simulink model "modeloProcessoAula4"  (R2022a)
settings: Solver=VariableStepAuto  StartTime=0.0  StopTime=400.0  RelTol=1e-3
values from neighbouring files (symbols this model uses):
  C = -14.405*(s + 0.0362)/s    [script.m]
  u0 = 52433    [script.m]
  y0 = 40982    [script.m]
libraries: cstblocks x5, slpidlib x1
settings Model: Creator=Victor  LastModifiedBy=Notebook_Artur
settings SolverCC: AlgebraicLoopSolver=TrustRegion
settings DebuggingCC: UnconnectedInputMsg=warning  UnconnectedOutputMsg=warning  UnconnectedLineMsg=warning  SFMachineParentedDataDiag=warning
settings RTWCC: DLArmComputeVersion=19.05

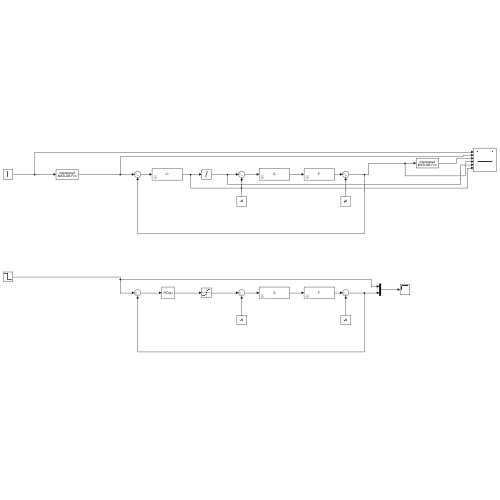
[thumbnail: Simulink's stored preview of the top-level diagram]
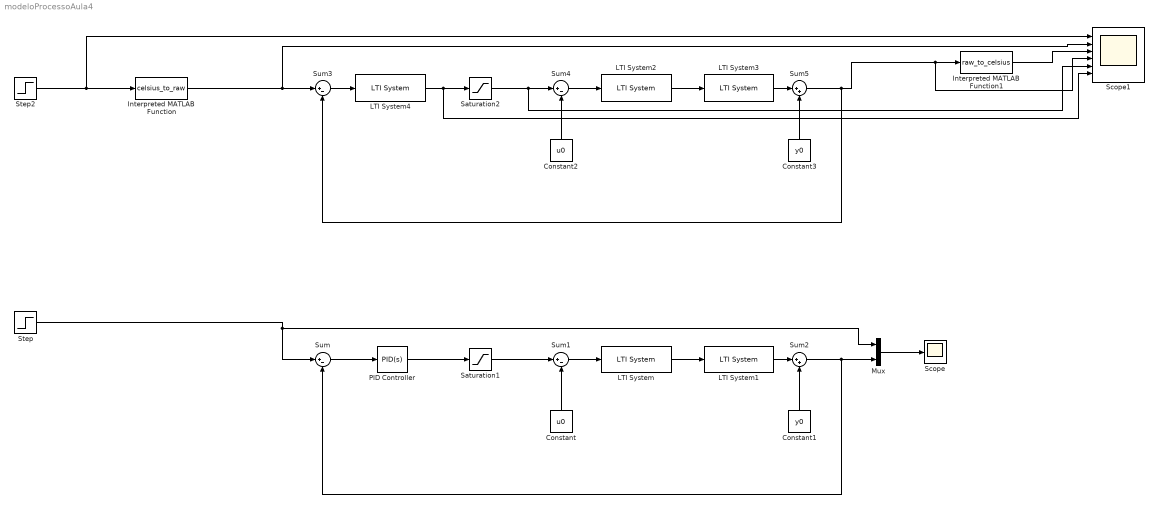
== system modeloProcessoAula4 ==
  Constant : Constant  Value=u0
  Constant1 : Constant  Value=y0
  Constant2 : Constant  Value=u0
  Constant3 : Constant  Value=y0
  Interpreted MATLAB Function : MATLABFcn  MATLABFcn=celsius_to_raw
  Interpreted MATLAB Function1 : MATLABFcn  MATLABFcn=raw_to_celsius
  LTI System : cstblocks/LTI System  sys=G  IC=[]
  LTI System1 : cstblocks/LTI System  sys=F  IC=[]
  LTI System2 : cstblocks/LTI System  sys=G  IC=[]
  LTI System3 : cstblocks/LTI System  sys=F  IC=[]
  LTI System4 : cstblocks/LTI System  sys=-C  IC=[]
  Mux : Mux  Inputs=2
  PID Controller : slpidlib/PID Controller  Controller=PID  Form=Parallel  TimeDomain=Continuous-time  UseExternalTs=off  SampleTime=-1  IntegratorMethod=Forward Euler  FilterMethod=Forward Euler  ControllerParametersSource=internal  P=11.5995607923269  I=0.355105773140582  UseKiTs=off  D=55.8366321204853  N=0.133857842452974  UseFilter=on  TunerSelectOption=Transfer Function Based (PID Tuner App)  InitialConditionSource=internal  InitialConditionForIntegrator=0  InitialConditionForFilter=0  DifferentiatorICPrevScaledInput=0  ExternalReset=none  TrackingMode=off  Kt=1  LimitOutput=off  SatLimitsSource=internal  UpperSaturationLimit=inf  LowerSaturationLimit=-inf  LinearizeAsGain=on  AntiWindupMode=none  Kb=1  POutMin=[]  POutMax=[]  IOutMin=[]  IOutMax=[]  DOutMin=[]  DOutMax=[]  NOutMin=[]  NOutMax=[]  SumOutMin=[]  SumOutMax=[]  SaturationOutMin=[]  SaturationOutMax=[]  PParamMin=[]  PParamMax=[]  IParamMin=[]  IParamMax=[]  DParamMin=[]  DParamMax=[]  NParamMin=[]  NParamMax=[]  KbParamMin=[]  KbParamMax=[]  KtParamMin=[]  KtParamMax=[]  KbOutMin=[]  KbOutMax=[]  KtOutMin=[]  KtOutMax=[]  IntegratorOutMin=[]  IntegratorOutMax=[]  FilterOutMin=[]  FilterOutMax=[]  SumI1OutMin=[]  SumI1OutMax=[]  SumI2OutMin=[]  SumI2OutMax=[]  SumI3OutMin=[]  SumI3OutMax=[]  SumI4OutMin=[]  SumI4OutMax=[]  SumDOutMin=[]  SumDOutMax=[]  DifferentiatorOutMin=[]  DifferentiatorOutMax=[]  FilterDiffOutCoefMin=[]  FilterDiffOutCoefMax=[]  ReciprocalOutMin=[]  ReciprocalOutMax=[]  SumDenOutMin=[]  SumDenOutMax=[]  SumNumOutMin=[]  SumNumOutMax=[]  DivideOutMin=[]  DivideOutMax=[]  UdiffTsProdOutMin=[]  UdiffTsProdOutMax=[]  NTsProdOutMin=[]  NTsProdOutMax=[]  UintegralTsProdOutMin=[]  UintegralTsProdOutMax=[]  UngainTsProdOutMin=[]  UngainTsProdOutMax=[]  IntegratorContinuousStateAttributes=''  IntegratorStateMustResolveToSignalObject=off  IntegratorRTWStateStorageClass=Auto  FilterContinuousStateAttributes=''  FilterStateMustResolveToSignalObject=off  FilterRTWStateStorageClass=Auto  ParallelPVariant=InternalParameters  IdealPVariant=Disabled  IVariant=InternalParameters  DVariant=InternalParameters  IntegratorVariant=Continuous  SatVariant=Disabled  AWVariant=Passthrough  PCopyVariant=Disabled  TRVariant=Disabled  FdbkBlocksVariant=Forward  IdealPFdbkVariant=Disabled  SatFdbkVariant=Disabled  DerivativeFilterVariant=ContFilter  NVariant=InternalParameters  NCopyVariant=Disabled  FilterICVariant=InternalICsFilter  IntegratorICVariant=InternalICs  ExternalResetVariant=Disabled  TRSumVariant=Passthrough  SumFdbkVariant=Disabled  SumVariant=Sum_PID  TsampFilterVariant=InternalTs  TsampNgainVariant=Passthrough  TsampIntegralVariant=Passthrough  ExternalSaturationOutDataTypeStr=Inherit: Same as second input  aMode=0
  Saturation1 : Saturate  UpperLimit=65535  LowerLimit=32786
  Saturation2 : Saturate  UpperLimit=65535  LowerLimit=32786
  Scope : Scope
  Scope1 : Scope  NumInputPorts=6
  Step : Step  Time=10  After=-6551  SampleTime=0
  Step2 : Step  Time=10  After=3  SampleTime=0
  Sum{,1,3..4} (4 alike) : Sum  Inputs=|+-
  Sum2 : Sum  Inputs=|++
  Sum5 : Sum  Inputs=|++
  wires:
  Constant/1 -> Sum1/2
  Constant1/1 -> Sum2/2
  Saturation1/1 -> Sum1/1
  Sum1/1 -> LTI System/1
  Sum2/1 -> Mux/2, Sum/2
  LTI System1/1 -> Sum2/1
  LTI System/1 -> LTI System1/1
  Step/1 -> Sum/1, Mux/1
  Mux/1 -> Scope/1
  Sum/1 -> PID Controller/1
  PID Controller/1 -> Saturation1/1
  Interpreted MATLAB Function/1 -> Scope1/2, Sum3/1
  LTI System3/1 -> Sum5/1
  Constant2/1 -> Sum4/2
  Sum5/1 -> Sum3/2, Scope1/4, Interpreted MATLAB Function1/1
  LTI System2/1 -> LTI System3/1
  Constant3/1 -> Sum5/2
  Saturation2/1 -> Scope1/5, Sum4/1
  Sum4/1 -> LTI System2/1
  LTI System4/1 -> Scope1/6, Saturation2/1
  Sum3/1 -> LTI System4/1
  Step2/1 -> Scope1/1, Interpreted MATLAB Function/1
  Interpreted MATLAB Function1/1 -> Scope1/3
